simulink model "IEEE68_BUS"  (R2019b)
settings: Solver=ode15s  StartTime=0.0  StopTime=10.0  FixedStep=Ts  RelTol=1e-3
PreLoadFcn:
  | Ts=50e-5;
  | 
  | % Required data to 68 Bus benchmark
  | % clear
  | % clc
  | % Definition for the columns
  | % system base =100 MVA
  | 
  | %% Line data Format (line)
  | % All values are given on the same system base MVA
  | % 1: From bus
  | % 2: To bus
  | % 3: Resistance (pu)
  | % 4: Reactance  (pu)
  | % 5: Charge     (pu)
  | % 6: Transformer Tap Amplitute
  | % 7: base MVA
  | % 8: Nomonal Voltage (KV)
  | 
  | %1   2    3        4       5       6        7      8
  | line=[...
  | 1	54	0	     0.0181	  0	      1.025     100    138
  | 2	58	0	     0.025	  0	      1.070     100    138
  | 3	62	0	     0.02	  0	      1.070     100    138
  | 4	19	0.0007	 0.0142	  0	      1.070     100    138
  | 5	20	0.0009	 0.018	  0	      1.009     100    138
  | 6	22	0	     0.0143	  0	      1.025     100    138
  | 7	23	0.0005	 0.0272	  0	      0         100    138
  | 8	25	0.0006	 0.0232	  0	      1.025     100    138
  | 9	29	0.0008	 0.0156   0	      1.025     100    138
  | 10	31	0	     0.026	  0	      1.04      100    138
  | 11	32	0	     0.013	  0	      1.04      100    138
  | 12	36	0	     0.0075	  0	      1.04      100    138
  | 13	17	0	     0.0033	  0	      1.04      100    138
  | 14	41	0	     0.0015	  0	      1         100    138
  | 15	42	0	     0.0015	  0	      1         100    138
  | 16	18	0	     0.003	  0	      1         100    138
  | 17	36	0.0005	 0.0045	  0.32	  0         100    138
  | 17	43	0.0005	 0.0276	  0	      0         100    138
  | 18	42	0.004	 0.06	  2.25    0         100    138
  | 18	49	0.0076	 0.1141	  1.16    0	        100    138
  | 18	50	0.0012	 0.0288	  2.06	  0         100    138
  | 20	19	0.0007	 0.0138	  0       1.06	    100    138
  | 19	68	0.0016	 0.0195	  0.304	  0         100    138
  | 21	22	0.0008	 0.014	  0.2565  0	        100    138
  | 21	68	0.0008	 0.0135	  0.2548  0	        100    138
  | 22	23	0.0006	 0.0096	  0.1846  0	        100    138
  | 23	24	0.0022	 0.035	  0.361	  0         100    138
  | 24	68	0.0003	 0.0059	  0.068	  0         100    138
  | 25	26	0.0032	 0.0323	  0.531	  0         100    138
  | 25	54	0.007	 0.0086	  0.146	  0         100    138
  | 26	27	0.0014	 0.0147	  0.2396  0	        100    138
  | 26	28	0.0043	 0.0474	  0.7802  0	        100    138
  | 26	29	0.0057	 0.0625	  1.029	  0         100    138
  | 27	37	0.0013	 0.0173	  0.3216  0	        100    138
  | 27	53	0.032	 0.32	  0.41	  0         100    138
  | 29	28	0.0014	 0.0151	  0.249	  0         100    138
  | 30	31	0.0013	 0.0187	  0.333	  0         100    138
  | 30	32	0.0024	 0.0288	  0.488	  0         100    138
  | 30	53	0.0008	 0.0074	  0.48	  0         100    138
  | ... (+201 lines)
InitFcn:
  | PSSMODEL=1;
  | LPSS=0;
  | WAPSS=0;
  | WAPSS2=0;
  | Ts=50e-5;
  | 
  | 
  | 
  | 
  | 
  | 
  | % Required data to 68 Bus benchmark
  | % clear
  | % clc
  | % Definition for the columns
  | % system base =100 MVA
  | 
  | %% Line data Format (line)
  | % All values are given on the same system base MVA
  | % 1: From bus
  | % 2: To bus
  | % 3: Resistance (pu)
  | % 4: Reactance  (pu)
  | % 5: Charge     (pu)
  | % 6: Transformer Tap Amplitute
  | % 7: base MVA
  | % 8: Nomonal Voltage (KV)
  | 
  | %1   2    3        4       5       6        7      8
  | line=[...
  | 1	54	0	     0.0181	  0	      1.025     100    138
  | 2	58	0	     0.025	  0	      1.070     100    138
  | 3	62	0	     0.02	  0	      1.070     100    138
  | 4	19	0.0007	 0.0142	  0	      1.070     100    138
  | 5	20	0.0009	 0.018	  0	      1.009     100    138
  | 6	22	0	     0.0143	  0	      1.025     100    138
  | 7	23	0.0005	 0.0272	  0	      0         100    138
  | 8	25	0.0006	 0.0232	  0	      1.025     100    138
  | 9	29	0.0008	 0.0156   0	      1.025     100    138
  | 10	31	0	     0.026	  0	      1.04      100    138
  | 11	32	0	     0.013	  0	      1.04      100    138
  | 12	36	0	     0.0075	  0	      1.04      100    138
  | 13	17	0	     0.0033	  0	      1.04      100    138
  | 14	41	0	     0.0015	  0	      1         100    138
  | 15	42	0	     0.0015	  0	      1         100    138
  | 16	18	0	     0.003	  0	      1         100    138
  | 17	36	0.0005	 0.0045	  0.32	  0         100    138
  | 17	43	0.0005	 0.0276	  0	      0         100    138
  | 18	42	0.004	 0.06	  2.25    0         100    138
  | 18	49	0.0076	 0.1141	  1.16    0	        100    138
  | 18	50	0.0012	 0.0288	  2.06	  0         100    138
  | 20	19	0.0007	 0.0138	  0       1.06	    100    138
  | 19	68	0.0016	 0.0195	  0.304	  0         100    138
  | 21	22	0.0008	 0.014	  0.2565  0	        100    138
  | 21	68	0.0008	 0.0135	  0.2548  0	        100    138
  | 22	23	0.0006	 0.0096	  0.1846  0	        100    138
  | 23	24	0.0022	 0.035	  0.361	  0         100    138
  | 24	68	0.0003	 0.0059	  0.068	  0         100    138
  | 25	26	0.0032	 0.0323	  0.531	  0         100    138
  | 25	54	0.007	 0.0086	  0.146	  0         100    138
  | ... (+185 lines)
undefined symbols (not defined in the file or in its folder): D1, Delta
libraries: powerlib x359, sps_avr x16, powerlib_meascontrol x5
(part 6 of 8)

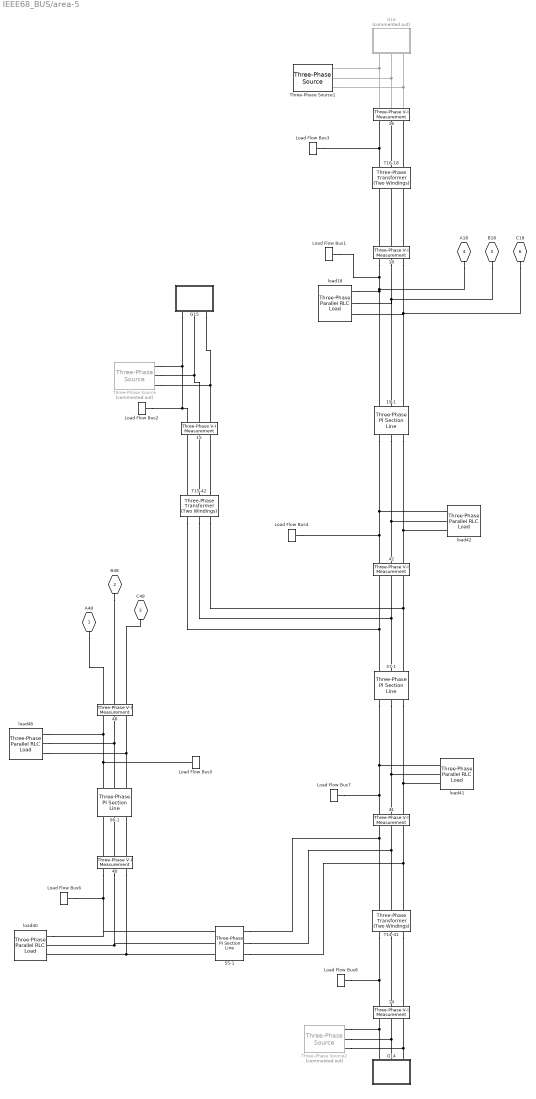
== system IEEE68_BUS/area-5 ==
  14 : powerlib/Measurements/Three-Phase V-I Measurement  VoltageMeasurement=phase-to-phase  SetLabelV=on  LabelV=Vabc_14  Vpu=off  VpuLL=on  CurrentMeasurement=no  SetLabelI=off  LabelI=Iabc  Ipu=off  Pbase=100e6  Vbase=13.8e3  OutputType=Complex  PhasorSimulation=on  PSBequivalent=0
      settings: SourceProductName=Simscape Electrical
  15 : powerlib/Measurements/Three-Phase V-I Measurement  VoltageMeasurement=phase-to-phase  SetLabelV=on  LabelV=Vabc_15  Vpu=off  VpuLL=on  CurrentMeasurement=no  SetLabelI=off  LabelI=Iabc  Ipu=off  Pbase=100e6  Vbase=13.8e3  OutputType=Complex  PhasorSimulation=on  PSBequivalent=0
      settings: SourceProductName=Simscape Electrical
  16 : powerlib/Measurements/Three-Phase V-I Measurement  VoltageMeasurement=phase-to-phase  SetLabelV=on  LabelV=Vabc_16  Vpu=off  VpuLL=on  CurrentMeasurement=no  SetLabelI=off  LabelI=Iabc  Ipu=off  Pbase=100e6  Vbase=13.8e3  OutputType=Complex  PhasorSimulation=on  PSBequivalent=0
      settings: SourceProductName=Simscape Electrical
  18 : powerlib/Measurements/Three-Phase V-I Measurement  VoltageMeasurement=phase-to-phase  SetLabelV=on  LabelV=Vabc_18  Vpu=off  VpuLL=on  CurrentMeasurement=no  SetLabelI=off  LabelI=Iabc  Ipu=off  Pbase=100e6  Vbase=Bus(18,2)*1e3  OutputType=Complex  PhasorSimulation=on  PSBequivalent=0
      settings: SourceProductName=Simscape Electrical
  19-1 : powerlib/Elements/Three-Phase PI Section Line  LConnTagsString=a|b|c  RConnTagsString=A|B|C  Frequency=60  Resistances=[line(19,3) 3*line(19,3)]  Inductances=[line(19,4) 3*line(19,4)]  Capacitances=[line(19,5) line(19,5)/3]  Length=1
      settings: SourceProductName=Simscape Electrical
  40 : powerlib/Measurements/Three-Phase V-I Measurement  VoltageMeasurement=phase-to-phase  SetLabelV=on  LabelV=Vabc_40  Vpu=off  VpuLL=on  CurrentMeasurement=no  SetLabelI=off  LabelI=Iabc  Ipu=off  Pbase=100e6  Vbase=Bus(40,2)*1e3  OutputType=Complex  PhasorSimulation=on  PSBequivalent=0
      settings: SourceProductName=Simscape Electrical
  41 : powerlib/Measurements/Three-Phase V-I Measurement  VoltageMeasurement=phase-to-phase  SetLabelV=on  LabelV=Vabc_41  Vpu=off  VpuLL=on  CurrentMeasurement=no  SetLabelI=off  LabelI=Iabc  Ipu=off  Pbase=100e6  Vbase=Bus(41,2)*1e3  OutputType=Complex  PhasorSimulation=on  PSBequivalent=0
      settings: SourceProductName=Simscape Electrical
  42 : powerlib/Measurements/Three-Phase V-I Measurement  VoltageMeasurement=phase-to-phase  SetLabelV=on  LabelV=Vabc_42  Vpu=off  VpuLL=on  CurrentMeasurement=no  SetLabelI=off  LabelI=Iabc  Ipu=off  Pbase=100e6  Vbase=Bus(42,2)*1e3  OutputType=Complex  PhasorSimulation=on  PSBequivalent=0
      settings: SourceProductName=Simscape Electrical
  48 : powerlib/Measurements/Three-Phase V-I Measurement  VoltageMeasurement=phase-to-phase  SetLabelV=on  LabelV=Vabc_48  Vpu=off  VpuLL=on  CurrentMeasurement=no  SetLabelI=off  LabelI=Iabc  Ipu=off  Pbase=100e6  Vbase=Bus(48,2)*1e3  OutputType=Complex  PhasorSimulation=on  PSBequivalent=0
      settings: SourceProductName=Simscape Electrical
  55-1 : powerlib/Elements/Three-Phase PI Section Line  LConnTagsString=a|b|c  RConnTagsString=A|B|C  Frequency=60  Resistances=[line(55,3) 3*line(55,3)]  Inductances=[line(55,4) 3*line(55,4)]  Capacitances=[line(55,5) line(55,5)/3]  Length=1
      settings: SourceProductName=Simscape Electrical
  56-1 : powerlib/Elements/Three-Phase PI Section Line  LConnTagsString=a|b|c  RConnTagsString=A|B|C  Frequency=60  Resistances=[line(56,3) 3*line(56,3)]  Inductances=[line(56,4) 3*line(56,4)]  Capacitances=[line(56,5) line(56,5)/3]  Length=1
      settings: SourceProductName=Simscape Electrical
  57-1 : powerlib/Elements/Three-Phase PI Section Line  LConnTagsString=a|b|c  RConnTagsString=A|B|C  Frequency=60  Resistances=[line(57,3) 3*line(57,3)]  Inductances=[line(57,4) 3*line(57,4)]  Capacitances=[line(57,5) line(57,5)/3]  Length=1
      settings: SourceProductName=Simscape Electrical
  G14 : Subsystem
  G15 : Subsystem
  G16 : Subsystem  Commented=on
  Load Flow Bus1 : powerlib/Measurements/Load Flow Bus  LConnTagsString=a  Phases=single  Connectors=on one side  ID=BUS_18  Vbase=138e03  Vref=1  Vangle=0  VLF=1  VLFb=1  VLFc=1  angleLF=0  angleLFb=0  angleLFc=0
      settings: SourceProductName=Simscape Electrical
  Load Flow Bus2 : powerlib/Measurements/Load Flow Bus  LConnTagsString=a  Phases=single  Connectors=on one side  ID=BUS_15  Vbase=13.8e03  Vref=1  Vangle=0  VLF=1  VLFb=1  VLFc=1  angleLF=0  angleLFb=0  angleLFc=0
      settings: SourceProductName=Simscape Electrical
  Load Flow Bus3 : powerlib/Measurements/Load Flow Bus  LConnTagsString=a  Phases=single  Connectors=on one side  ID=BUS_16  Vbase=13.8e03  Vref=1  Vangle=0  VLF=1  VLFb=1  VLFc=1  angleLF=0  angleLFb=0  angleLFc=0
      settings: SourceProductName=Simscape Electrical
  Load Flow Bus4 : powerlib/Measurements/Load Flow Bus  LConnTagsString=a  Phases=single  Connectors=on one side  ID=BUS_42  Vbase=138e03  Vref=1  Vangle=0  VLF=1  VLFb=1  VLFc=1  angleLF=0  angleLFb=0  angleLFc=0
      settings: SourceProductName=Simscape Electrical
  Load Flow Bus5 : powerlib/Measurements/Load Flow Bus  LConnTagsString=a  Phases=single  Connectors=on one side  ID=BUS_48  Vbase=138e03  Vref=1  Vangle=0  VLF=1  VLFb=1  VLFc=1  angleLF=0  angleLFb=0  angleLFc=0
      settings: SourceProductName=Simscape Electrical
  Load Flow Bus6 : powerlib/Measurements/Load Flow Bus  LConnTagsString=a  Phases=single  Connectors=on one side  ID=BUS_40  Vbase=138e03  Vref=1  Vangle=0  VLF=1  VLFb=1  VLFc=1  angleLF=0  angleLFb=0  angleLFc=0
      settings: SourceProductName=Simscape Electrical
  Load Flow Bus7 : powerlib/Measurements/Load Flow Bus  LConnTagsString=a  Phases=single  Connectors=on one side  ID=BUS_41  Vbase=138e03  Vref=1  Vangle=0  VLF=1  VLFb=1  VLFc=1  angleLF=0  angleLFb=0  angleLFc=0
      settings: SourceProductName=Simscape Electrical
  Load Flow Bus8 : powerlib/Measurements/Load Flow Bus  LConnTagsString=a  Phases=single  Connectors=on one side  ID=BUS_14  Vbase=13.8e03  Vref=1  Vangle=0  VLF=1  VLFb=1  VLFc=1  angleLF=0  angleLFb=0  angleLFc=0
      settings: SourceProductName=Simscape Electrical
  T14-41 : powerlib/Elements/Three-Phase Transformer (Two Windings)  Winding1Connection=Delta (D1)  Winding2Connection=Yg  CoreType=Three single-phase transformers  SetSaturation=off  Hysteresis=off  DataFile='hysteresis'  SetInitialFlux=off  Measurements=None  UNITS=pu  NominalPower=[ 10000e6 , 60 ]  Winding1=[ 13.8e3 , 0.0002 , 0 ]  Winding2=[ 138e3 , 0.0002 , 0.0015 ]  Rm=500  Lm=500  L0=0.5  Saturation=[ 0,0 ; 0.0024,1.2 ; 1.0,1.52 ]  InitialFluxes=[ 0.8 , -0.8 , 0.7 ]  BreakLoop=off  DiscreteSolver=Trapezoidal robust  DataType=off  TransfoNumber=1
      settings: SourceProductName=Simscape Electrical
  T15-42 : powerlib/Elements/Three-Phase Transformer (Two Windings)  Winding1Connection=Delta (D1)  Winding2Connection=Yg  CoreType=Three single-phase transformers  SetSaturation=off  Hysteresis=off  DataFile='hysteresis'  SetInitialFlux=off  Measurements=None  UNITS=pu  NominalPower=[ 10000e6 , 60 ]  Winding1=[ 13.8e3 , 0.0002 , 0 ]  Winding2=[ 138e3 , 0.0002, 0.0015 ]  Rm=500  Lm=500  L0=0.5  Saturation=[ 0,0 ; 0.0024,1.2 ; 1.0,1.52 ]  InitialFluxes=[ 0.8 , -0.8 , 0.7 ]  BreakLoop=off  DiscreteSolver=Trapezoidal robust  DataType=off  TransfoNumber=1
      settings: SourceProductName=Simscape Electrical
  T16-18 : powerlib/Elements/Three-Phase Transformer (Two Windings)  Winding1Connection=Delta (D1)  Winding2Connection=Yg  CoreType=Three single-phase transformers  SetSaturation=off  Hysteresis=off  DataFile='hysteresis'  SetInitialFlux=off  Measurements=None  UNITS=pu  NominalPower=[ 10000e6 , 60 ]  Winding1=[ 13.8e3 , 0.0002 , 0 ]  Winding2=[ 138e3 , 0.0002, 0.0015 ]  Rm=500  Lm=500  L0=0.5  Saturation=[ 0,0 ; 0.0024,1.2 ; 1.0,1.52 ]  InitialFluxes=[ 0.8 , -0.8 , 0.7 ]  BreakLoop=off  DiscreteSolver=Trapezoidal robust  DataType=off  TransfoNumber=1
      settings: SourceProductName=Simscape Electrical
  Three-Phase Source : powerlib/Electrical Sources/Three-Phase Source  Commented=on  InternalConnection=Yg  VoltagePhases=off  Voltage=138e3  PhaseAngle=0  Voltage_phases=[25e3 25e3 25e3]/sqrt(3)  PhaseAngles_phases=[0 -120 +120]  Frequency=60  NonIdealSource=on  SpecifyImpedance=off  Resistance=0.8929  Inductance=16.58e-3  ShortCircuitLevel=100e6  BaseVoltage=138e3  XRratio=7  BusType=PV  Pref=1000e6  Qref=0  Prefabc=[10e3, 10e3, 10e3]  Qrefabc=[0, 0, 0]  Qmin=-inf  Qmax=inf
      settings: SourceProductName=Simscape Electrical
  Three-Phase Source1 : powerlib/Electrical Sources/Three-Phase Source  InternalConnection=Yg  VoltagePhases=off  Voltage=13.8e3  PhaseAngle=0  Voltage_phases=[25e3 25e3 25e3]/sqrt(3)  PhaseAngles_phases=[0 -120 +120]  Frequency=60  NonIdealSource=on  SpecifyImpedance=on  Resistance=0.8929  Inductance=16.58e-3  ShortCircuitLevel=3500e6  BaseVoltage=13.8e3  XRratio=7  BusType=swing  Pref=1000e6  Qref=0  Prefabc=[10e3, 10e3, 10e3]  Qrefabc=[0, 0, 0]  Qmin=-inf  Qmax=inf
      settings: SourceProductName=Simscape Electrical
  Three-Phase Source2 : powerlib/Electrical Sources/Three-Phase Source  Commented=on  InternalConnection=Yg  VoltagePhases=off  Voltage=138e3  PhaseAngle=0  Voltage_phases=[25e3 25e3 25e3]/sqrt(3)  PhaseAngles_phases=[0 -120 +120]  Frequency=60  NonIdealSource=on  SpecifyImpedance=off  Resistance=0.8929  Inductance=16.58e-3  ShortCircuitLevel=100e6  BaseVoltage=138e3  XRratio=7  BusType=PV  Pref=1785e6  Qref=0  Prefabc=[10e3, 10e3, 10e3]  Qrefabc=[0, 0, 0]  Qmin=-inf  Qmax=inf
      settings: SourceProductName=Simscape Electrical
  load18 : powerlib/Elements/Three-Phase Parallel RLC Load  LConnTagsString=A|B|C  Configuration=Y (grounded)  NominalVoltage=138000  Vabc=[1e3 1e3 1e3]  Vabcp=[1e3 1e3 1e3]  NominalFrequency=60  UnbalancedPower=off  ActivePower=2470e6  InductivePower=123e6  CapacitivePower=0  Pabc=[10e3 9e3 11e3]  QLabc=[100 90 110]  QCabc=[100 90 110]  Pabcp=[10e3 9e3 11e3]  QLabcp=[100 90 110]  QCabcp=[100 90 110]  Measurements=None  LoadType=constant PQ
      settings: SourceProductName=Simscape Electrical
  load40 : powerlib/Elements/Three-Phase Parallel RLC Load  LConnTagsString=A|B|C  Configuration=Y (grounded)  NominalVoltage=138000  Vabc=[1e3 1e3 1e3]  Vabcp=[1e3 1e3 1e3]  NominalFrequency=60  UnbalancedPower=off  ActivePower=66e6  InductivePower=24e6  CapacitivePower=0  Pabc=[10e3 9e3 11e3]  QLabc=[100 90 110]  QCabc=[100 90 110]  Pabcp=[10e3 9e3 11e3]  QLabcp=[100 90 110]  QCabcp=[100 90 110]  Measurements=None  LoadType=constant PQ
      settings: SourceProductName=Simscape Electrical
  load41 : powerlib/Elements/Three-Phase Parallel RLC Load  LConnTagsString=A|B|C  Configuration=Y (grounded)  NominalVoltage=138000  Vabc=[1e3 1e3 1e3]  Vabcp=[1e3 1e3 1e3]  NominalFrequency=60  UnbalancedPower=off  ActivePower=1000e6  InductivePower=250e6  CapacitivePower=0  Pabc=[10e3 9e3 11e3]  QLabc=[100 90 110]  QCabc=[100 90 110]  Pabcp=[10e3 9e3 11e3]  QLabcp=[100 90 110]  QCabcp=[100 90 110]  Measurements=None  LoadType=constant PQ
      settings: SourceProductName=Simscape Electrical
  load42 : powerlib/Elements/Three-Phase Parallel RLC Load  LConnTagsString=A|B|C  Configuration=Y (grounded)  NominalVoltage=138000  Vabc=[1e3 1e3 1e3]  Vabcp=[1e3 1e3 1e3]  NominalFrequency=60  UnbalancedPower=off  ActivePower=1150e6  InductivePower=250e6  CapacitivePower=0  Pabc=[10e3 9e3 11e3]  QLabc=[100 90 110]  QCabc=[100 90 110]  Pabcp=[10e3 9e3 11e3]  QLabcp=[100 90 110]  QCabcp=[100 90 110]  Measurements=None  LoadType=constant PQ
      settings: SourceProductName=Simscape Electrical
  load48 : powerlib/Elements/Three-Phase Parallel RLC Load  LConnTagsString=A|B|C  Configuration=Y (grounded)  NominalVoltage=138000  Vabc=[1e3 1e3 1e3]  Vabcp=[1e3 1e3 1e3]  NominalFrequency=60  UnbalancedPower=off  ActivePower=241e6  InductivePower=2e6  CapacitivePower=0  Pabc=[10e3 9e3 11e3]  QLabc=[100 90 110]  QCabc=[100 90 110]  Pabcp=[10e3 9e3 11e3]  QLabcp=[100 90 110]  QCabcp=[100 90 110]  Measurements=None  LoadType=constant PQ
      settings: SourceProductName=Simscape Electrical
  A48 : PMIOPort  Tag=PMCPort  Side=Right
  B48 : PMIOPort  Tag=PMCPort  Port=2  Side=Right
  C48 : PMIOPort  Tag=PMCPort  Port=3  Side=Right
  A18 : PMIOPort  Tag=PMCPort  Port=4  Side=Right
  B18 : PMIOPort  Tag=PMCPort  Port=5  Side=Right
  C18 : PMIOPort  Tag=PMCPort  Port=6  Side=Right
  connections:
  40/RConn2 -- 56-1/LConn2
  56-1/RConn3 -- load48/LConn3 -- 48/LConn3
  40/RConn3 -- 56-1/LConn3
  56-1/RConn1 -- Load Flow Bus5/LConn1 -- load48/LConn1 -- 48/LConn1
  40/RConn1 -- 56-1/LConn1
  56-1/RConn2 -- load48/LConn2 -- 48/LConn2
  G14/LConn1 -- Three-Phase Source2/RConn1 -- 14/RConn1
  G14/LConn2 -- Three-Phase Source2/RConn2 -- 14/RConn2
  G14/LConn3 -- Three-Phase Source2/RConn3 -- 14/RConn3
  T14-41/RConn1 -- 55-1/RConn1 -- 41/RConn1
  T14-41/RConn2 -- 55-1/RConn2 -- 41/RConn2
  T14-41/RConn3 -- 55-1/RConn3 -- 41/RConn3
  T14-41/LConn1 -- Load Flow Bus8/LConn1 -- 14/LConn1
  T14-41/LConn2 -- 14/LConn2
  T14-41/LConn3 -- 14/LConn3
  40/LConn1 -- 55-1/LConn1 -- load40/LConn1 -- Load Flow Bus6/LConn1
  40/LConn2 -- 55-1/LConn2 -- load40/LConn2
  40/LConn3 -- load40/LConn3 -- 55-1/LConn3
  57-1/LConn1 -- T15-42/RConn1 -- 42/RConn1
  57-1/LConn2 -- T15-42/RConn2 -- 42/RConn2
  57-1/LConn3 -- T15-42/RConn3 -- 42/RConn3
  57-1/RConn1 -- Load Flow Bus7/LConn1 -- 41/LConn1 -- load41/LConn1
  57-1/RConn2 -- load41/LConn2 -- 41/LConn2
  57-1/RConn3 -- load41/LConn3 -- 41/LConn3
  19-1/RConn1 -- load42/LConn1 -- Load Flow Bus4/LConn1 -- 42/LConn1
  19-1/RConn2 -- 42/LConn2 -- load42/LConn2
  19-1/RConn3 -- 42/LConn3 -- load42/LConn3
  G15/LConn1 -- Three-Phase Source/RConn1 -- 15/RConn1 -- Load Flow Bus2/LConn1
  G15/LConn2 -- Three-Phase Source/RConn2 -- 15/RConn2
  G15/LConn3 -- Three-Phase Source/RConn3 -- 15/RConn3
  T15-42/LConn1 -- 15/LConn1
  T15-42/LConn2 -- 15/LConn2
  T15-42/LConn3 -- 15/LConn3
  G16/LConn1 -- Three-Phase Source1/RConn1 -- 16/RConn1
  G16/LConn2 -- Three-Phase Source1/RConn2 -- 16/RConn2
  G16/LConn3 -- Three-Phase Source1/RConn3 -- 16/RConn3
  T16-18/LConn1 -- 16/LConn1 -- Load Flow Bus3/LConn1
  T16-18/LConn2 -- 16/LConn2
  T16-18/LConn3 -- 16/LConn3
  A48/RConn1 -- 48/RConn1
  B48/RConn1 -- 48/RConn2
  C48/RConn1 -- 48/RConn3
  18/RConn3 -- T16-18/RConn3
  18/RConn2 -- T16-18/RConn2
  18/RConn1 -- T16-18/RConn1
  18/LConn1 -- Load Flow Bus1/LConn1 -- A18/RConn1 -- load18/LConn1 -- 19-1/LConn1
  18/LConn2 -- load18/LConn2 -- 19-1/LConn2 -- B18/RConn1
  18/LConn3 -- load18/LConn3 -- 19-1/LConn3 -- C18/RConn1

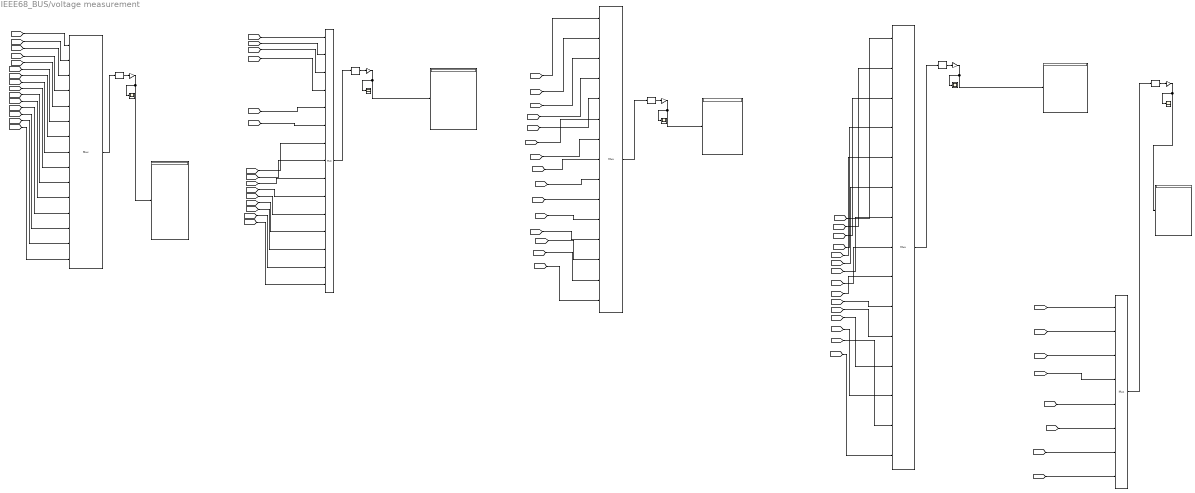
== system IEEE68_BUS/voltage measurement  ==
  Display{,1..4} (5 alike) : Display
  Gain{1..4} (4 alike) : Gain  Gain=2*sqrt(2)/sqrt(3)
  Gain5 : Gain  Gain=2/sqrt(3)
  Mux{1..4} (4 alike) : Mux  Inputs=15
  Mux5 : Mux  Inputs=8
  RMS{1..5} (5 alike) : powerlib_meascontrol/Measurements/RMS  TrueRMS=on  Freq=60  RMSInit=120  Ts=Ts
      settings: SourceProductName=Simscape Electrical
  Scope{1..5} (5 alike) : Scope
  wires:
  Mux1/1 -> RMS2/1
  [Vabc_05] -> Mux1/5
  [Vabc_06] -> Mux1/6
  Gain2/1 -> Display/1, Scope1/1
  [Vabc_03] -> Mux1/3
  [Vabc_11] -> Mux1/11
  [Vabc_10] -> Mux1/10
  [Vabc_07] -> Mux1/7
  [Vabc_09] -> Mux1/9
  [Vabc_01] -> Mux1/1
  [Vabc_13] -> Mux1/13
  [Vabc_02] -> Mux1/2
  [Vabc_12] -> Mux1/12
  [Vabc_14] -> Mux1/14
  [Vabc_08] -> Mux1/8
  RMS2/1 -> Gain2/1
  [Vabc_04] -> Mux1/4
  [Vabc_15] -> Mux1/15
  Mux2/1 -> RMS1/1
  RMS1/1 -> Gain1/1
  Gain1/1 -> Scope2/1, Display1/1
  [Vabc_16] -> Mux2/1
  [Vabc_17] -> Mux2/2
  [Vabc_18] -> Mux2/3
  Gain3/1 -> Scope3/1, Display2/1
  RMS3/1 -> Gain3/1
  Mux3/1 -> RMS3/1
  Gain4/1 -> Scope4/1, Display3/1
  RMS4/1 -> Gain4/1
  Mux4/1 -> RMS4/1
  [Vabc_19] -> Mux2/4
  [Vabc_20] -> Mux2/5
  [Vabc_21] -> Mux2/6
  [Vabc_22] -> Mux2/7
  [Vabc_23] -> Mux2/8
  [Vabc_24] -> Mux2/9
  [Vabc_25] -> Mux2/10
  [Vabc_26] -> Mux2/11
  [Vabc_27] -> Mux2/12
  [Vabc_28] -> Mux2/13
  [Vabc_29] -> Mux2/14
  [Vabc_30] -> Mux2/15
  [Vabc_31] -> Mux3/1
  [Vabc_32] -> Mux3/2
  [Vabc_33] -> Mux3/3
  [Vabc_34] -> Mux3/4
  [Vabc_35] -> Mux3/5
  [Vabc_36] -> Mux3/6
  [Vabc_37] -> Mux3/7
  [Vabc_38] -> Mux3/8
  [Vabc_39] -> Mux3/9
  [Vabc_40] -> Mux3/10
  [Vabc_41] -> Mux3/11
  [Vabc_42] -> Mux3/12
  [Vabc_43] -> Mux3/13
  [Vabc_44] -> Mux3/14
  [Vabc_45] -> Mux3/15
  [Vabc_46] -> Mux4/1
  [Vabc_47] -> Mux4/2
  [Vabc_48] -> Mux4/3
  [Vabc_49] -> Mux4/4
  [Vabc_50] -> Mux4/5
  [Vabc_51] -> Mux4/6
  [Vabc_52] -> Mux4/7
  [Vabc_53] -> Mux4/8
  [Vabc_54] -> Mux4/9
  [Vabc_55] -> Mux4/10
  [Vabc_56] -> Mux4/11
  [Vabc_57] -> Mux4/12
  [Vabc_58] -> Mux4/13
  [Vabc_59] -> Mux4/14
  [Vabc_60] -> Mux4/15
  Gain5/1 -> Display4/1, Scope5/1
  RMS5/1 -> Gain5/1
  Mux5/1 -> RMS5/1
  [Vabc_61] -> Mux5/1
  [Vabc_62] -> Mux5/2
  [Vabc_63] -> Mux5/3
  [Vabc_64] -> Mux5/4
  [Vabc_65] -> Mux5/5
  [Vabc_66] -> Mux5/6
  [Vabc_67] -> Mux5/7
  [Vabc_68] -> Mux5/8

== system IEEE68_BUS/area-1/gen4 ==
  "M4: Turbine & Regulators " : Subsystem
  Pref4 : Constant  Value=0.7
  Synchronous Machine SI Fundamental : powerlib/Machines/Synchronous Machine SI Fundamental  Commented=on  PresetModel=No  MechanicalLoad=Mechanical power Pm  ShowDetailedParameters=on  RotorType=Salient-pole  Units=SI fundamental parameters  MeasurementBus=off  NominalParameters="[ 187E6  13800   60   1087 ]"  Stator="[ 2.9069E-03  3.0892E-04  3.2164E-03  9.7153E-04 ]"  Field="[ 5.9013E-04  3.0712E-04 ]"  Dampers2=[ 0.0664, 1.387e-3, 0.0292, 6.896e-4, 7.907e-3, 2.477e-3]  Dampers1="[ 1.1900E-02  4.9076E-04  2.0081E-02  1.0365E-03 ]"  Mechanical=[ 3.895e6 0 20 ]  PolePairs=20  InitialConditions="[ 0  0  0  0  0  0  0  0  70.3192 ]"  SetSaturation=off  Saturation=[695.64,774.7,917.5,1001.6,1082.2,1175.9,1293.6,1430.2,1583.7;9660,10623,12243,13063,13757,14437,15180,15890,16567]  DisplayVfd=off  LoadFlowParameters=[1,0,0,0,0]  TsPowergui=0  TsBlock=-1  IterativeModel=Trapezoidal non iterative  IterativeDiscreteModel=Trapezoidal non iterative  BusType=PV  Pref=0  Qref=0  Qmin=-inf  Qmax=inf  PLF=0  QLF=0
      settings: SourceProductName=Simscape Electrical  SourceProductBaseCode=PS
  Synchronous Machine pu Standard : powerlib/Machines/Synchronous Machine pu Standard  Commented=on  PresetModel=No  MechanicalLoad=Mechanical power Pm  ShowDetailedParameters=on  RotorType=Salient-pole  Units=per unit standard parameters  MeasurementBus=off  NominalParameters=[6e+04 400 50]  Reactances1=[ 1.81, 0.3, 0.23, 1.76, 0.65, 0.25, 0.15 ]  Reactances2=[2.24 0.17 0.12 1.02 0.13 0.08]  dAxisTimeConstants=Short-circuit  qAxisTimeConstants=Short-circuit  TimeConstants1="[ 4.4849  0.0681  0.1  ]"  TimeConstants2=[ 8.0, 0.03, 1.0, 0.07 ]  TimeConstants3="[  4.49  0.0681  0.0513  ]"  TimeConstants4=[ 8.0, 0.03, 0.3371, 0.0295 ]  TimeConstants5=[ 1.01, 0.053, 0.1 ]  TimeConstants6=[ 1.3201, 0.023, 1.0, 0.07 ]  TimeConstants7=[0.012 0.003 0.003]  TimeConstants8=[ 1.3201, 0.0231, 0.3371, 0.0295 ]  StatorResistance=0.037875  Mechanical=[0.1028 0.02056 2]  PolePairs=20  InitialConditions="[ 0  0  0  0  0  0  0  0  1 ]"  SetSaturation=on  Saturation=[0.6404,0.7127,0.8441,0.9214,0.9956,1.082,1.19,1.316,1.457;0.7,0.7698,0.8872,0.9466,0.9969,1.046,1.1,1.151,1.201]  LoadFlowParameters=[1,0,0,0,0]  TsPowergui=0  TsBlock=-1  IterativeModel=Trapezoidal non iterative  IterativeDiscreteModel=Trapezoidal non iterative  BusType=PV  Pref=0  Qref=0  Qmin=-inf  Qmax=inf  PLF=0  QLF=0
      settings: SourceProductName=Simscape Electrical
  Vref4 : Constant  Value=0.997
  gen4 : powerlib/Machines/Synchronous Machine pu Standard  PresetModel=No  MechanicalLoad=Mechanical power Pm  ShowDetailedParameters=on  RotorType=Round  Units=per unit standard parameters  MeasurementBus=off  NominalParameters="[1000*1e6  13.8*1e3   60 ]"  Reactances1="[mac_con(4,6:8)  mac_con(4,11:13)  mac_con(4,4)]"  Reactances2=[ 1.305, 0.296, 0.252, 0.474, 0.243, 0.18 ]  dAxisTimeConstants=Open-circuit  qAxisTimeConstants=Open-circuit  TimeConstants1=[]  TimeConstants2="[mac_con(4,9:10)  mac_con(4,14:15)]"  TimeConstants3=[]  TimeConstants4=[]  TimeConstants5=[ 1.01, 0.053, 0.1 ]  TimeConstants6=[]  TimeConstants7=[]  TimeConstants8=[]  StatorResistance=mac_con(4,5)  Mechanical="[ mac_con(4,16)  0  4]"  PolePairs=4  InitialConditions=[0 -27.7466 0.647548 0.647548 0.647548 -0.416201 -120.416 119.584 2.14879]  SetSaturation=off  Saturation=[0.6404,0.7127,0.8441,0.9214,0.9956,1.082,1.19,1.316,1.457;0.7,0.7698,0.8872,0.9466,0.9969,1.046,1.1,1.151,1.201]  LoadFlowParameters=[1 830000000 0 0 0]  TsPowergui=0  TsBlock=-1  IterativeModel=Trapezoidal non iterative  IterativeDiscreteModel=Trapezoidal non iterative  BusType=PV  Pref=632e6  Qref=0  Qmin=-inf  Qmax=inf  PLF=0  QLF=0
      settings: AttributesFormatString=\n\n  SourceProductName=Simscape Electrical
  A : PMIOPort  Side=Left
  B : PMIOPort  Port=2  Side=Left
  C : PMIOPort  Port=3  Side=Left
  wires:
  Pref4/1 -> "M4: Turbine & Regulators "/2(Pref4)
  "M4: Turbine & Regulators "/1(Pm4) -> gen4/1
  "M4: Turbine & Regulators "/2(Vf4) -> gen4/2
  gen4/1 -> "M4: Turbine & Regulators "/1(m4)
  [PSSmodel] -> "M4: Turbine & Regulators "/4(PSS4)
  Vref4/1 -> "M4: Turbine & Regulators "/3(Vref4)
  connections:
  A/RConn1 -- gen4/RConn1
  B/RConn1 -- gen4/RConn2
  C/RConn1 -- gen4/RConn3

== system IEEE68_BUS/area-1/gen5 ==
  "M4: Turbine & Regulators " : Subsystem
  Pref5 : Constant  Value=0.7
  Vref5 : Constant  Value=1.011
  gen5 : powerlib/Machines/Synchronous Machine pu Standard  PresetModel=No  MechanicalLoad=Mechanical power Pm  ShowDetailedParameters=on  RotorType=Round  Units=per unit standard parameters  MeasurementBus=off  NominalParameters="[1000*1e6  13.8e3   60 ]"  Reactances1="[mac_con(5,6:8)  mac_con(5,11:13)  mac_con(5,4)]"  Reactances2=[ 1.305, 0.296, 0.252, 0.474, 0.243, 0.18 ]  dAxisTimeConstants=Open-circuit  qAxisTimeConstants=Open-circuit  TimeConstants1=[]  TimeConstants2="[mac_con(5,9:10)  mac_con(5,14:15)]"  TimeConstants3=[]  TimeConstants4=[]  TimeConstants5=[ 1.01, 0.053, 0.1 ]  TimeConstants6=[]  TimeConstants7=[]  TimeConstants8=[]  StatorResistance=mac_con(5,5)  Mechanical="[ mac_con(5,16)  0  4]"  PolePairs=4  InitialConditions=[0 -18.657 0.524928 0.524928 0.524928 -3.22796 -123.228 116.772 3.89055]  SetSaturation=off  Saturation=[0.6404,0.7127,0.8441,0.9214,0.9956,1.082,1.19,1.316,1.457;0.7,0.7698,0.8872,0.9466,0.9969,1.046,1.1,1.151,1.201]  LoadFlowParameters=[1 830000000 0 0 0]  TsPowergui=0  TsBlock=-1  IterativeModel=Trapezoidal non iterative  IterativeDiscreteModel=Trapezoidal non iterative  BusType=PV  Pref=505e6  Qref=0  Qmin=-inf  Qmax=inf  PLF=0  QLF=0
      settings: AttributesFormatString=\n\n  SourceProductName=Simscape Electrical
  A : PMIOPort  Side=Left
  B : PMIOPort  Port=2  Side=Left
  C : PMIOPort  Port=3  Side=Left
  wires:
  Vref5/1 -> "M4: Turbine & Regulators "/3(Vref5)
  [PSSmodel] -> "M4: Turbine & Regulators "/4(PSS4)
  gen5/1 -> "M4: Turbine & Regulators "/1(m5)
  "M4: Turbine & Regulators "/2(Vf5) -> gen5/2
  "M4: Turbine & Regulators "/1(Pm4) -> gen5/1
  Pref5/1 -> "M4: Turbine & Regulators "/2(Pref5)
  connections:
  C/RConn1 -- gen5/RConn3
  B/RConn1 -- gen5/RConn2
  A/RConn1 -- gen5/RConn1

== system IEEE68_BUS/area-1/gen6 ==
  "M4: Turbine & Regulators " : Subsystem
  Pref6 : Constant  Value=0.8
  Synchronous Machine SI Fundamental : powerlib/Machines/Synchronous Machine SI Fundamental  Commented=on  PresetModel=No  MechanicalLoad=Mechanical power Pm  ShowDetailedParameters=on  RotorType=Salient-pole  Units=SI fundamental parameters  MeasurementBus=off  NominalParameters="[ 187E6  13800   60   1087 ]"  Stator="[ 2.9069E-03  3.0892E-04  3.2164E-03  9.7153E-04 ]"  Field="[ 5.9013E-04  3.0712E-04 ]"  Dampers2=[ 0.0664, 1.387e-3, 0.0292, 6.896e-4, 7.907e-3, 2.477e-3]  Dampers1="[ 1.1900E-02  4.9076E-04  2.0081E-02  1.0365E-03 ]"  Mechanical=[ 3.895e6 0 20 ]  PolePairs=20  InitialConditions="[ 0  0  0  0  0  0  0  0  70.3192 ]"  SetSaturation=off  Saturation=[695.64,774.7,917.5,1001.6,1082.2,1175.9,1293.6,1430.2,1583.7;9660,10623,12243,13063,13757,14437,15180,15890,16567]  DisplayVfd=off  LoadFlowParameters=[1,0,0,0,0]  TsPowergui=0  TsBlock=-1  IterativeModel=Trapezoidal non iterative  IterativeDiscreteModel=Trapezoidal non iterative  BusType=PV  Pref=0  Qref=0  Qmin=-inf  Qmax=inf  PLF=0  QLF=0
      settings: SourceProductName=Simscape Electrical  SourceProductBaseCode=PS
  Synchronous Machine pu Standard : powerlib/Machines/Synchronous Machine pu Standard  Commented=on  PresetModel=No  MechanicalLoad=Mechanical power Pm  ShowDetailedParameters=on  RotorType=Salient-pole  Units=per unit standard parameters  MeasurementBus=off  NominalParameters=[6e+04 400 50]  Reactances1=[ 1.81, 0.3, 0.23, 1.76, 0.65, 0.25, 0.15 ]  Reactances2=[2.24 0.17 0.12 1.02 0.13 0.08]  dAxisTimeConstants=Short-circuit  qAxisTimeConstants=Short-circuit  TimeConstants1="[ 4.4849  0.0681  0.1  ]"  TimeConstants2=[ 8.0, 0.03, 1.0, 0.07 ]  TimeConstants3="[  4.49  0.0681  0.0513  ]"  TimeConstants4=[ 8.0, 0.03, 0.3371, 0.0295 ]  TimeConstants5=[ 1.01, 0.053, 0.1 ]  TimeConstants6=[ 1.3201, 0.023, 1.0, 0.07 ]  TimeConstants7=[0.012 0.003 0.003]  TimeConstants8=[ 1.3201, 0.0231, 0.3371, 0.0295 ]  StatorResistance=0.037875  Mechanical=[0.1028 0.02056 2]  PolePairs=20  InitialConditions="[ 0  0  0  0  0  0  0  0  1 ]"  SetSaturation=on  Saturation=[0.6404,0.7127,0.8441,0.9214,0.9956,1.082,1.19,1.316,1.457;0.7,0.7698,0.8872,0.9466,0.9969,1.046,1.1,1.151,1.201]  LoadFlowParameters=[1,0,0,0,0]  TsPowergui=0  TsBlock=-1  IterativeModel=Trapezoidal non iterative  IterativeDiscreteModel=Trapezoidal non iterative  BusType=PV  Pref=0  Qref=0  Qmin=-inf  Qmax=inf  PLF=0  QLF=0
      settings: SourceProductName=Simscape Electrical
  Vref6 : Constant  Value=1.05
  gen6 : powerlib/Machines/Synchronous Machine pu Standard  PresetModel=No  MechanicalLoad=Mechanical power Pm  ShowDetailedParameters=on  RotorType=Round  Units=per unit standard parameters  MeasurementBus=off  NominalParameters="[1000*1e6  13.8*1e3   60 ]"  Reactances1="[mac_con(4,6:8)  mac_con(4,11:13)  mac_con(4,4)]"  Reactances2=[ 1.305, 0.296, 0.252, 0.474, 0.243, 0.18 ]  dAxisTimeConstants=Open-circuit  qAxisTimeConstants=Open-circuit  TimeConstants1=[]  TimeConstants2="[mac_con(4,9:10)  mac_con(4,14:15)]"  TimeConstants3=[]  TimeConstants4=[]  TimeConstants5=[ 1.01, 0.053, 0.1 ]  TimeConstants6=[]  TimeConstants7=[]  TimeConstants8=[]  StatorResistance=mac_con(4,5)  Mechanical="[ mac_con(4,16)  0  4]"  PolePairs=4  InitialConditions=[0 -27.7466 0.647548 0.647548 0.647548 -0.416201 -120.416 119.584 2.14879]  SetSaturation=off  Saturation=[0.6404,0.7127,0.8441,0.9214,0.9956,1.082,1.19,1.316,1.457;0.7,0.7698,0.8872,0.9466,0.9969,1.046,1.1,1.151,1.201]  LoadFlowParameters=[1 830000000 0 0 0]  TsPowergui=0  TsBlock=-1  IterativeModel=Trapezoidal non iterative  IterativeDiscreteModel=Trapezoidal non iterative  BusType=PV  Pref=700e6  Qref=0  Qmin=-inf  Qmax=inf  PLF=0  QLF=0
      settings: AttributesFormatString=\n\n  SourceProductName=Simscape Electrical
  A : PMIOPort  Side=Left
  B : PMIOPort  Port=2  Side=Left
  C : PMIOPort  Port=3  Side=Left
  wires:
  Vref6/1 -> "M4: Turbine & Regulators "/3(Vref6)
  [PSSmodel] -> "M4: Turbine & Regulators "/4(PSS6)
  gen6/1 -> "M4: Turbine & Regulators "/1(m6)
  "M4: Turbine & Regulators "/2(Vf6) -> gen6/2
  "M4: Turbine & Regulators "/1(Pm6) -> gen6/1
  Pref6/1 -> "M4: Turbine & Regulators "/2(Pref6)
  connections:
  C/RConn1 -- gen6/RConn3
  B/RConn1 -- gen6/RConn2
  A/RConn1 -- gen6/RConn1

== system IEEE68_BUS/area-1/gen7 ==
  "M7: Turbine & Regulators " : Subsystem
  Pref7 : Constant  Value=0.7
  Synchronous Machine SI Fundamental : powerlib/Machines/Synchronous Machine SI Fundamental  Commented=on  PresetModel=No  MechanicalLoad=Mechanical power Pm  ShowDetailedParameters=on  RotorType=Salient-pole  Units=SI fundamental parameters  MeasurementBus=off  NominalParameters="[ 187E6  13800   60   1087 ]"  Stator="[ 2.9069E-03  3.0892E-04  3.2164E-03  9.7153E-04 ]"  Field="[ 5.9013E-04  3.0712E-04 ]"  Dampers2=[ 0.0664, 1.387e-3, 0.0292, 6.896e-4, 7.907e-3, 2.477e-3]  Dampers1="[ 1.1900E-02  4.9076E-04  2.0081E-02  1.0365E-03 ]"  Mechanical=[ 3.895e6 0 20 ]  PolePairs=20  InitialConditions="[ 0  0  0  0  0  0  0  0  70.3192 ]"  SetSaturation=off  Saturation=[695.64,774.7,917.5,1001.6,1082.2,1175.9,1293.6,1430.2,1583.7;9660,10623,12243,13063,13757,14437,15180,15890,16567]  DisplayVfd=off  LoadFlowParameters=[1,0,0,0,0]  TsPowergui=0  TsBlock=-1  IterativeModel=Trapezoidal non iterative  IterativeDiscreteModel=Trapezoidal non iterative  BusType=PV  Pref=0  Qref=0  Qmin=-inf  Qmax=inf  PLF=0  QLF=0
      settings: SourceProductName=Simscape Electrical  SourceProductBaseCode=PS
  Synchronous Machine pu Standard : powerlib/Machines/Synchronous Machine pu Standard  Commented=on  PresetModel=No  MechanicalLoad=Mechanical power Pm  ShowDetailedParameters=on  RotorType=Salient-pole  Units=per unit standard parameters  MeasurementBus=off  NominalParameters=[6e+04 400 50]  Reactances1=[ 1.81, 0.3, 0.23, 1.76, 0.65, 0.25, 0.15 ]  Reactances2=[2.24 0.17 0.12 1.02 0.13 0.08]  dAxisTimeConstants=Short-circuit  qAxisTimeConstants=Short-circuit  TimeConstants1="[ 4.4849  0.0681  0.1  ]"  TimeConstants2=[ 8.0, 0.03, 1.0, 0.07 ]  TimeConstants3="[  4.49  0.0681  0.0513  ]"  TimeConstants4=[ 8.0, 0.03, 0.3371, 0.0295 ]  TimeConstants5=[ 1.01, 0.053, 0.1 ]  TimeConstants6=[ 1.3201, 0.023, 1.0, 0.07 ]  TimeConstants7=[0.012 0.003 0.003]  TimeConstants8=[ 1.3201, 0.0231, 0.3371, 0.0295 ]  StatorResistance=0.037875  Mechanical=[0.1028 0.02056 2]  PolePairs=20  InitialConditions="[ 0  0  0  0  0  0  0  0  1 ]"  SetSaturation=on  Saturation=[0.6404,0.7127,0.8441,0.9214,0.9956,1.082,1.19,1.316,1.457;0.7,0.7698,0.8872,0.9466,0.9969,1.046,1.1,1.151,1.201]  LoadFlowParameters=[1,0,0,0,0]  TsPowergui=0  TsBlock=-1  IterativeModel=Trapezoidal non iterative  IterativeDiscreteModel=Trapezoidal non iterative  BusType=PV  Pref=0  Qref=0  Qmin=-inf  Qmax=inf  PLF=0  QLF=0
      settings: SourceProductName=Simscape Electrical
  Vref7 : Constant  Value=1.06
  gen7 : powerlib/Machines/Synchronous Machine pu Standard  PresetModel=No  MechanicalLoad=Mechanical power Pm  ShowDetailedParameters=on  RotorType=Round  Units=per unit standard parameters  MeasurementBus=off  NominalParameters="[1000*1e6  138*1e3   60 ]"  Reactances1="[mac_con(4,6:8)  mac_con(4,11:13)  mac_con(4,4)]"  Reactances2=[ 1.305, 0.296, 0.252, 0.474, 0.243, 0.18 ]  dAxisTimeConstants=Open-circuit  qAxisTimeConstants=Open-circuit  TimeConstants1=[]  TimeConstants2="[mac_con(4,9:10)  mac_con(4,14:15)]"  TimeConstants3=[]  TimeConstants4=[]  TimeConstants5=[ 1.01, 0.053, 0.1 ]  TimeConstants6=[]  TimeConstants7=[]  TimeConstants8=[]  StatorResistance=mac_con(4,5)  Mechanical="[ mac_con(4,16)  0  4]"  PolePairs=4  InitialConditions=[0 -27.7466 0.647548 0.647548 0.647548 -0.416201 -120.416 119.584 2.14879]  SetSaturation=off  Saturation=[0.6404,0.7127,0.8441,0.9214,0.9956,1.082,1.19,1.316,1.457;0.7,0.7698,0.8872,0.9466,0.9969,1.046,1.1,1.151,1.201]  LoadFlowParameters=[1 830000000 0 0 0]  TsPowergui=0  TsBlock=-1  IterativeModel=Trapezoidal non iterative  IterativeDiscreteModel=Trapezoidal non iterative  BusType=PV  Pref=560e6  Qref=0  Qmin=-inf  Qmax=inf  PLF=0  QLF=0
      settings: AttributesFormatString=\n\n  SourceProductName=Simscape Electrical
  A : PMIOPort  Side=Left
  B : PMIOPort  Port=2  Side=Left
  C : PMIOPort  Port=3  Side=Left
  wires:
  Vref7/1 -> "M7: Turbine & Regulators "/3(Vref7)
  [PSSmodel] -> "M7: Turbine & Regulators "/4(PSS7)
  gen7/1 -> "M7: Turbine & Regulators "/1(m7)
  "M7: Turbine & Regulators "/2(Vf7) -> gen7/2
  "M7: Turbine & Regulators "/1(Pm7) -> gen7/1
  Pref7/1 -> "M7: Turbine & Regulators "/2(Pref7)
  connections:
  C/RConn1 -- gen7/RConn3
  B/RConn1 -- gen7/RConn2
  A/RConn1 -- gen7/RConn1

== system IEEE68_BUS/area-2/G2 ==
  2 : Constant  Value=0.98
  "M2: Turbine & Regulators " : Subsystem
  Pref2 : Constant  Value=0.545
  gen2 : powerlib/Machines/Synchronous Machine pu Standard  PresetModel=No  MechanicalLoad=Mechanical power Pm  ShowDetailedParameters=on  RotorType=Round  Units=per unit standard parameters  MeasurementBus=off  NominalParameters="[1000*1e6  13.8e3   60 ]"  Reactances1="[mac_con(2,6:8)  mac_con(2,11:13)  mac_con(2,4)]"  Reactances2=[ 1.305, 0.296, 0.252, 0.474, 0.243, 0.18 ]  dAxisTimeConstants=Open-circuit  qAxisTimeConstants=Open-circuit  TimeConstants1=[]  TimeConstants2="[mac_con(2,9:10)  mac_con(2,14:15)]"  TimeConstants3=[]  TimeConstants4=[]  TimeConstants5=[ 1.01, 0.053, 0.1 ]  TimeConstants6=[]  TimeConstants7=[]  TimeConstants8=[]  StatorResistance=mac_con(2,5)  Mechanical="[ mac_con(2,16)  0  4]"  PolePairs=4  InitialConditions=[0 -63.2657 0.339533 0.339533 0.339533 -35.2425 -155.242 84.7575 1.77729]  SetSaturation=off  Saturation=[0.6404,0.7127,0.8441,0.9214,0.9956,1.082,1.19,1.316,1.457;0.7,0.7698,0.8872,0.9466,0.9969,1.046,1.1,1.151,1.201]  LoadFlowParameters=[1 830000000 0 0 0]  TsPowergui=0  TsBlock=-1  IterativeModel=Trapezoidal non iterative  IterativeDiscreteModel=Trapezoidal non iterative  BusType=PV  Pref=545*1e6  Qref=0  Qmin=-inf  Qmax=inf  PLF=0  QLF=0
      settings: AttributesFormatString=\n\n  SourceProductName=Simscape Electrical
  A : PMIOPort  Side=Left
  B : PMIOPort  Port=2  Side=Left
  C : PMIOPort  Port=3  Side=Left
  wires:
  Pref2/1 -> "M2: Turbine & Regulators "/2(Pref2)
  "M2: Turbine & Regulators "/1(Pm2) -> gen2/1
  "M2: Turbine & Regulators "/2(Vf2) -> gen2/2
  gen2/1 -> "M2: Turbine & Regulators "/1(m2)
  [PSSmodel] -> "M2: Turbine & Regulators "/4(PSS2)
  2/1 -> "M2: Turbine & Regulators "/3(Vref2)
  connections:
  A/RConn1 -- gen2/RConn1
  B/RConn1 -- gen2/RConn2
  C/RConn1 -- gen2/RConn3

== system IEEE68_BUS/area-2/gen3 ==
  "M3: Turbine & Regulators " : Subsystem
  Pref3 : Constant  Value=0.7
  Vref3 : Constant  Value=0.983
  gen3 : powerlib/Machines/Synchronous Machine pu Standard  PresetModel=No  MechanicalLoad=Mechanical power Pm  ShowDetailedParameters=on  RotorType=Round  Units=per unit standard parameters  MeasurementBus=off  NominalParameters="[2000*1e6  13.8e3   60 ]"  Reactances1="[mac_con(3,6:8)  mac_con(3,11:13)  mac_con(3,4)]"  Reactances2=[ 1.305, 0.296, 0.252, 0.474, 0.243, 0.18 ]  dAxisTimeConstants=Open-circuit  qAxisTimeConstants=Open-circuit  TimeConstants1=[]  TimeConstants2="[mac_con(3,9:10)  mac_con(3,14:15)]"  TimeConstants3=[]  TimeConstants4=[]  TimeConstants5=[ 1.01, 0.053, 0.1 ]  TimeConstants6=[]  TimeConstants7=[]  TimeConstants8=[]  StatorResistance=mac_con(3,5)  Mechanical="[ mac_con(3,16)  0  4]"  PolePairs=4  InitialConditions=[0 -37.958 0.689466 0.689466 0.689466 -12.356 -132.356 107.644 2.25944]  SetSaturation=off  Saturation=[0.6404,0.7127,0.8441,0.9214,0.9956,1.082,1.19,1.316,1.457;0.7,0.7698,0.8872,0.9466,0.9969,1.046,1.1,1.151,1.201]  LoadFlowParameters=[1 830000000 0 0 0]  TsPowergui=0  TsBlock=-1  IterativeModel=Trapezoidal non iterative  IterativeDiscreteModel=Trapezoidal non iterative  BusType=PV  Pref=650*1e6  Qref=0  Qmin=-inf  Qmax=inf  PLF=0  QLF=0
      settings: AttributesFormatString=\n\n  SourceProductName=Simscape Electrical
  A : PMIOPort  Side=Left
  B : PMIOPort  Port=2  Side=Left
  C : PMIOPort  Port=3  Side=Left
  wires:
  Vref3/1 -> "M3: Turbine & Regulators "/3(Vref3)
  [PSSmodel] -> "M3: Turbine & Regulators "/4(PSS3)
  gen3/1 -> "M3: Turbine & Regulators "/1(m3)
  "M3: Turbine & Regulators "/2(Vf3) -> gen3/2
  "M3: Turbine & Regulators "/1(Pm3) -> gen3/1
  Pref3/1 -> "M3: Turbine & Regulators "/2(Pref3)
  connections:
  C/RConn1 -- gen3/RConn3
  B/RConn1 -- gen3/RConn2
  A/RConn1 -- gen3/RConn1

== system IEEE68_BUS/area-3/G1 ==
  "M1: Turbine & Regulators " : Subsystem
  Pref1 : Constant  Value=0.25
  Vref1 : Constant  Value=1.045
  gen1 : powerlib/Machines/Synchronous Machine pu Standard  PresetModel=No  MechanicalLoad=Mechanical power Pm  ShowDetailedParameters=on  RotorType=Round  Units=per unit standard parameters  MeasurementBus=off  NominalParameters="[1000*1e6  13.8e3  60 ]"  Reactances1="[mac_con(1,6:8)  mac_con(1,11:13)  mac_con(1,4)]"  Reactances2=[ 1.305, 0.296, 0.252, 0.474, 0.243, 0.18 ]  dAxisTimeConstants=Open-circuit  qAxisTimeConstants=Open-circuit  TimeConstants1=[]  TimeConstants2="[mac_con(1,9:10)  mac_con(1,14:15)]"  TimeConstants3=[]  TimeConstants4=[]  TimeConstants5=[ 1.01, 0.053, 0.1 ]  TimeConstants6=[]  TimeConstants7=[]  TimeConstants8=[]  StatorResistance=mac_con(1,5)  Mechanical="[ mac_con(1,16)  0  4]"  PolePairs=4  InitialConditions=[0 -53.3817 1.03438 1.03438 1.03438 11.5505 -108.45 131.55 1.07168]  SetSaturation=off  Saturation=[0.6404,0.7127,0.8441,0.9214,0.9956,1.082,1.19,1.316,1.457;0.7,0.7698,0.8872,0.9466,0.9969,1.046,1.1,1.151,1.201]  LoadFlowParameters=[1 830000000 0 0 0]  TsPowergui=0  TsBlock=-1  IterativeModel=Trapezoidal non iterative  IterativeDiscreteModel=Trapezoidal non iterative  BusType=PV  Pref=250*1e6  Qref=0  Qmin=-inf  Qmax=inf  PLF=0  QLF=0
      settings: AttributesFormatString=\n\n  SourceProductName=Simscape Electrical
  A : PMIOPort  Side=Left
  B : PMIOPort  Port=2  Side=Left
  C : PMIOPort  Port=3  Side=Left
  wires:
  Vref1/1 -> "M1: Turbine & Regulators "/3(Vref1)
  [PSSmodel] -> "M1: Turbine & Regulators "/4(PSS1)
  gen1/1 -> "M1: Turbine & Regulators "/1(m1)
  "M1: Turbine & Regulators "/2(Vf1) -> gen1/2
  "M1: Turbine & Regulators "/1(Pm1) -> gen1/1
  Pref1/1 -> "M1: Turbine & Regulators "/2(Pref1)
  connections:
  C/RConn1 -- gen1/RConn3
  B/RConn1 -- gen1/RConn2
  A/RConn1 -- gen1/RConn1

== system IEEE68_BUS/area-3/G8 ==
  "M8: Turbine & Regulators " : Subsystem
  Pref8 : Constant  Value=0.54
  Vref8 : Constant  Value=1.03
  gen8 : powerlib/Machines/Synchronous Machine pu Standard  PresetModel=No  MechanicalLoad=Mechanical power Pm  ShowDetailedParameters=on  RotorType=Round  Units=per unit standard parameters  MeasurementBus=off  NominalParameters="[1000*1e6  13.8e3   60 ]"  Reactances1="[mac_con(8,6:8)  mac_con(8,11:13)  mac_con(8,4)]"  Reactances2=[ 1.305, 0.296, 0.252, 0.474, 0.243, 0.18 ]  dAxisTimeConstants=Open-circuit  qAxisTimeConstants=Open-circuit  TimeConstants1=[]  TimeConstants2="[mac_con(8,9:10)  mac_con(8,14:15)]"  TimeConstants3=[]  TimeConstants4=[]  TimeConstants5=[ 1.01, 0.053, 0.1 ]  TimeConstants6=[]  TimeConstants7=[]  TimeConstants8=[]  StatorResistance=mac_con(8,5)  Mechanical="[ mac_con(8,16)  0  4]"  PolePairs=4  InitialConditions=[0 -25.6939 0.5409 0.5409 0.5409 6.7214 -113.279 126.721 1.90805]  SetSaturation=off  Saturation=[0.6404,0.7127,0.8441,0.9214,0.9956,1.082,1.19,1.316,1.457;0.7,0.7698,0.8872,0.9466,0.9969,1.046,1.1,1.151,1.201]  LoadFlowParameters=[1 830000000 0 0 0]  TsPowergui=0  TsBlock=-1  IterativeModel=Trapezoidal non iterative  IterativeDiscreteModel=Trapezoidal non iterative  BusType=PV  Pref=540*1e6  Qref=0  Qmin=-inf  Qmax=inf  PLF=0  QLF=0
      settings: AttributesFormatString=\n\n  SourceProductName=Simscape Electrical
  A : PMIOPort  Side=Left
  B : PMIOPort  Port=2  Side=Left
  C : PMIOPort  Port=3  Side=Left
  wires:
  Pref8/1 -> "M8: Turbine & Regulators "/2(Pref8)
  "M8: Turbine & Regulators "/1(Pm8) -> gen8/1
  "M8: Turbine & Regulators "/2(Vf8) -> gen8/2
  gen8/1 -> "M8: Turbine & Regulators "/1(m8)
  [PSSmodel] -> "M8: Turbine & Regulators "/4(PSS8)
  Vref8/1 -> "M8: Turbine & Regulators "/3(Vref8)
  connections:
  A/RConn1 -- gen8/RConn1
  B/RConn1 -- gen8/RConn2
  C/RConn1 -- gen8/RConn3

== system IEEE68_BUS/area-3/G9 ==
  "M9: Turbine & Regulators " : Subsystem
  Pref9 : Constant  Value=0.9
  Vref9 : Constant  Value=1.025
  gen9 : powerlib/Machines/Synchronous Machine pu Standard  PresetModel=No  MechanicalLoad=Mechanical power Pm  ShowDetailedParameters=on  RotorType=Round  Units=per unit standard parameters  MeasurementBus=off  NominalParameters="[1000*1e6  13.8e3   60 ]"  Reactances1="[mac_con(9,6:8)  mac_con(9,11:13)  mac_con(9,4)]"  Reactances2=[ 1.305, 0.296, 0.252, 0.474, 0.243, 0.18 ]  dAxisTimeConstants=Open-circuit  qAxisTimeConstants=Open-circuit  TimeConstants1=[]  TimeConstants2="[mac_con(9,9:10)  mac_con(9,14:15)]"  TimeConstants3=[]  TimeConstants4=[]  TimeConstants5=[ 1.01, 0.053, 0.1 ]  TimeConstants6=[]  TimeConstants7=[]  TimeConstants8=[]  StatorResistance=mac_con(9,5)  Mechanical="[ mac_con(9,16)  0  4]"  PolePairs=4  InitialConditions=[0 -16.7125 0.832308 0.832308 0.832308 12.5378 -107.462 132.538 2.08155]  SetSaturation=off  Saturation=[0.6404,0.7127,0.8441,0.9214,0.9956,1.082,1.19,1.316,1.457;0.7,0.7698,0.8872,0.9466,0.9969,1.046,1.1,1.151,1.201]  LoadFlowParameters=[1 830000000 0 0 0]  TsPowergui=0  TsBlock=-1  IterativeModel=Trapezoidal non iterative  IterativeDiscreteModel=Trapezoidal non iterative  BusType=PV  Pref=800*1e6  Qref=0  Qmin=-inf  Qmax=inf  PLF=0  QLF=0
      settings: AttributesFormatString=\n\n  SourceProductName=Simscape Electrical
  A : PMIOPort  Side=Left
  B : PMIOPort  Port=2  Side=Left
  C : PMIOPort  Port=3  Side=Left
  wires:
  Vref9/1 -> "M9: Turbine & Regulators "/3(Vref9)
  [PSSmodel] -> "M9: Turbine & Regulators "/4(PSS9)
  gen9/1 -> "M9: Turbine & Regulators "/1(m9)
  "M9: Turbine & Regulators "/2(Vf9) -> gen9/2
  "M9: Turbine & Regulators "/1(Pm9) -> gen9/1
  Pref9/1 -> "M9: Turbine & Regulators "/2(Pref9)
  connections:
  C/RConn1 -- gen9/RConn3
  B/RConn1 -- gen9/RConn2
  A/RConn1 -- gen9/RConn1

== system IEEE68_BUS/area-4/G10 ==
  "M10: Turbine & Regulators " : Subsystem
  Pref10 : Constant  Value=0.6
  Vref10 : Constant  Value=1.01
  gen10 : powerlib/Machines/Synchronous Machine pu Standard  PresetModel=No  MechanicalLoad=Mechanical power Pm  ShowDetailedParameters=on  RotorType=Round  Units=per unit standard parameters  MeasurementBus=off  NominalParameters="[1000*1e6  13.8e3   60 ]"  Reactances1="[mac_con(10,6:8)  mac_con(10,11:13)  mac_con(10,4)]"  Reactances2=[ 1.305, 0.296, 0.252, 0.474, 0.243, 0.18 ]  dAxisTimeConstants=Open-circuit  qAxisTimeConstants=Open-circuit  TimeConstants1=[]  TimeConstants2="[mac_con(10,9:10)  mac_con(10,14:15)]"  TimeConstants3=[]  TimeConstants4=[]  TimeConstants5=[ 1.01, 0.053, 0.1 ]  TimeConstants6=[]  TimeConstants7=[]  TimeConstants8=[]  StatorResistance=mac_con(10,5)  Mechanical="[ mac_con(10,16)  0  4]"  PolePairs=4  InitialConditions=[0 -76.9944 0.265611 0.265611 0.265611 -15.9627 -135.963 104.037 1.1157]  SetSaturation=off  Saturation=[0.6404,0.7127,0.8441,0.9214,0.9956,1.082,1.19,1.316,1.457;0.7,0.7698,0.8872,0.9466,0.9969,1.046,1.1,1.151,1.201]  LoadFlowParameters=[1 830000000 0 0 0]  TsPowergui=0  TsBlock=-1  IterativeModel=Trapezoidal non iterative  IterativeDiscreteModel=Trapezoidal non iterative  BusType=PV  Pref=500*1e6  Qref=0  Qmin=-inf  Qmax=inf  PLF=0  QLF=0
      settings: AttributesFormatString=\n\n  SourceProductName=Simscape Electrical
  A : PMIOPort  Side=Left
  B : PMIOPort  Port=2  Side=Left
  C : PMIOPort  Port=3  Side=Left
  wires:
  Vref10/1 -> "M10: Turbine & Regulators "/3(Vref10)
  [PSSmodel] -> "M10: Turbine & Regulators "/4(PSS10)
  gen10/1 -> "M10: Turbine & Regulators "/1(m10)
  "M10: Turbine & Regulators "/2(Vf10) -> gen10/2
  "M10: Turbine & Regulators "/1(Pm10) -> gen10/1
  Pref10/1 -> "M10: Turbine & Regulators "/2(Pref10)
  connections:
  C/RConn1 -- gen10/RConn3
  B/RConn1 -- gen10/RConn2
  A/RConn1 -- gen10/RConn1
